simulink subsystem "s0518_swing_fast3"  (R2019b)
settings: Solver=VariableStepAuto  StartTime=0.0  StopTime=10.0  RelTol=1e-3
settings Model: Creator=Student  LastModifiedBy=giaco

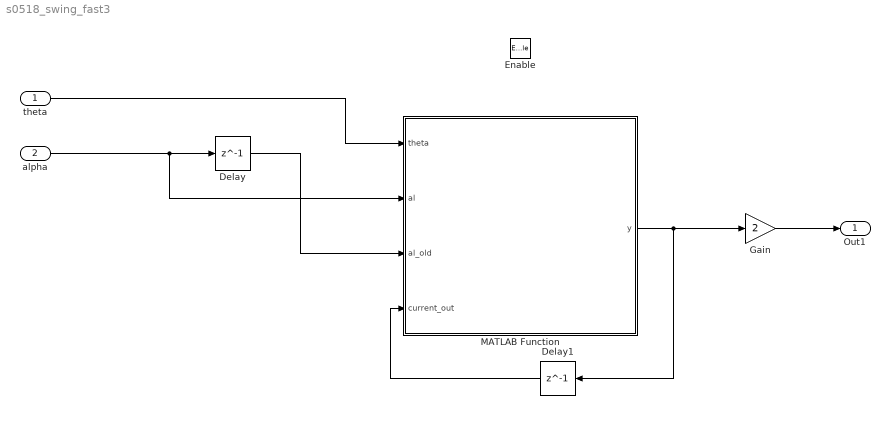
== system s0518_swing_fast3 ==
  theta : Inport
  alpha : Inport  Port=2
  Enable : EnablePort  StatesWhenEnabling=reset
  Delay : Delay  DelayLength=1  InitialCondition=0
  Delay1 : Delay  DelayLength=1  InitialCondition=1
  Gain : Gain  Gain=2
  MATLAB Function : MATLAB Function  TreatAsAtomicUnit=on
  Out1 : Outport
  wires:
  Delay1/1 -> MATLAB Function/4(current_out)
  Gain/1 -> Out1/1
  Delay/1 -> MATLAB Function/3(al_old)
  alpha/1 -> Delay/1, MATLAB Function/2(al)
  theta/1 -> MATLAB Function/1(theta)
  MATLAB Function/1(y) -> Delay1/1, Gain/1

== matlab function s0518_swing_fast3/MATLAB Function ==
  data: theta input; y output; al input; al_old input; current_out input
function y = fcn(theta, al, al_old, current_out)

stop_condition = false;
while ~stop_condition
    if al > pi
        al = al - 2*pi;
    elseif al < -pi
        al = al + 2*pi;
    else
        stop_condition = true;
    end
end

stop_condition = false;
while ~stop_condition
    if al_old > pi
        al_old = al_old - 2*pi;
    elseif al_old < -pi
        al_old = al_old + 2*pi;
    else
        stop_condition = true;
    end
end


if abs(al) < pi/2 && al < al_old && current_out == 1
    
    signum = -1;
    
elseif abs(al) < pi/2 && al > al_old && current_out == -1
    
    signum = 1;
    
elseif abs(al) >= pi/2 && al < al_old && current_out == -1
    
    signum = 1;
    
elseif abs(al) >= pi/2 && al > al_old && current_out == 1
    
    signum = -1;
    
elseif abs(al) >= pi/2 && abs(al_old)<pi/2
    
    signum = -current_out;
    
else
    signum = current_out;
    
end
    
if theta > pi/4 && signum == 1
    
    signum = -1;
    
elseif theta < -pi/4 && signum == -1
    
    signum = 1;
    
end

y = signum;
